simulink model "ofdm4"  (R2018b)
settings: Solver=VariableStepAuto  StartTime=0.0  StopTime=10.0  RelTol=1e-3
undefined symbols (not defined in the file or in its folder): doppler
libraries: commrandsrc3 x3, commutil2 x2, simulink x2, dspmathops x2, commdigbbndpm3 x2, commofdm x2, commrflib2 x2, commfilt2 x2, commdigbbndam3 x2, commsink2 x1, commchan3 x1
settings Model: Creator=Aviya  LastModifiedBy=Aviya

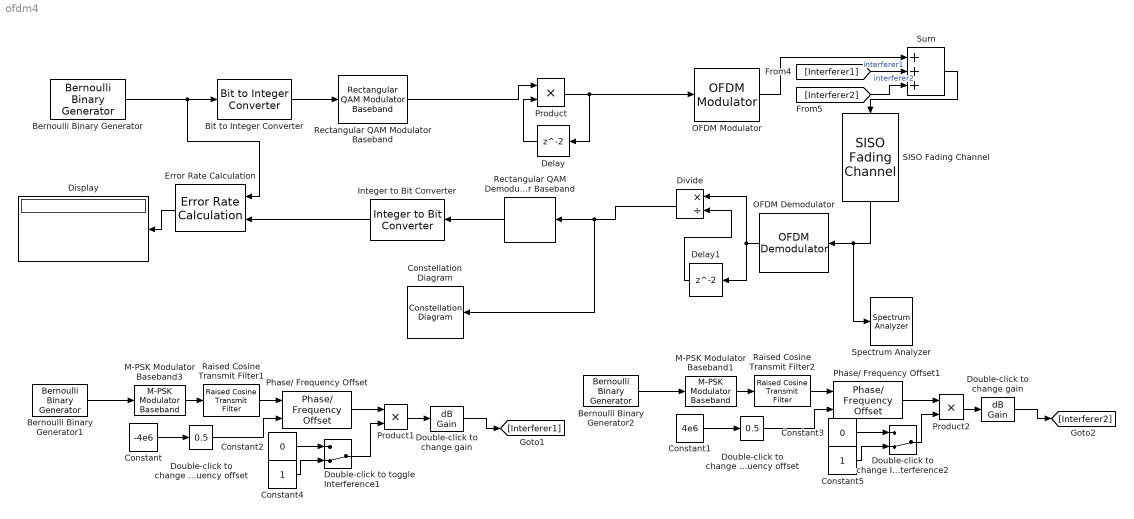
== system ofdm4 ==
  Bernoulli Binary Generator : commrandsrc3/Bernoulli Binary Generator  ProbabilityOfZero=0.5  SeedSource=Parameter  Seed=61  SampleTime=1  SamplesPerFrame=53  OutputDataType=double  SimulateUsing=Interpreted execution
      settings: SourceProductName=Communications Toolbox
  Bernoulli Binary Generator1 : commrandsrc3/Bernoulli Binary Generator  ProbabilityOfZero=0.5  SeedSource=Parameter  Seed=61  SampleTime=1  SamplesPerFrame=80  OutputDataType=boolean  SimulateUsing=Interpreted execution
  Bernoulli Binary Generator2 : commrandsrc3/Bernoulli Binary Generator  ProbabilityOfZero=0.5  SeedSource=Parameter  Seed=61  SampleTime=1  SamplesPerFrame=80  OutputDataType=boolean  SimulateUsing=Interpreted execution
  Bit to Integer Converter : commutil2/Bit to Integer Converter  nbits=1  bitOrder=MSB first  signedOutputValues=Unsigned  outDtype=single  outDtypeSigned=Inherit via internal rule
      settings: SourceProductName=Communications Toolbox
  Constant : Constant  Value=-4e6  VectorParams1D=off  SampleTime=(1e-6/3)*300
  Constant1 : Constant  Value=4e6  VectorParams1D=off  SampleTime=(1e-6/3)*300
  Constant2 : Constant  Value=0  VectorParams1D=off  SampleTime=(1e-6/3)*300
  Constant3 : Constant  Value=0  VectorParams1D=off  SampleTime=(1e-6/3)*300
  Constant4 : Constant  VectorParams1D=off  SampleTime=(1e-6/3)*300
  Constant5 : Constant  VectorParams1D=off  SampleTime=(1e-6/3)*300
  Constellation Diagram : ConstellationDiagram
  Delay : Delay
  Delay1 : Delay
  Display : Display
  Divide : Product  Inputs=*/
  Double-click to change Interference2 : ManualSwitch  CurrentSetting=0
  Double-click to change frequency offset : simulink/Math Operations/Slider Gain  gain=0.5  low=-0.85  high=0.85
  Double-click to change gain : dspmathops/dB Gain  dB=-20  intype=Amplitude
      settings: SourceProductName=DSP System Toolbox  SourceProductBaseCode=DS
  "Double-click to change gain " : dspmathops/dB Gain  dB=-10  intype=Amplitude
      settings: SourceProductName=DSP System Toolbox  SourceProductBaseCode=DS
  Double-click to toggle Interference1 : ManualSwitch  CurrentSetting=0
  Double-click to change frequency offset : simulink/Math Operations/Slider Gain  gain=0.5  low=-0.85  high=0.85
  Error Rate Calculation : commsink2/Error Rate Calculation  N=0  st_delay=0  cp_mode=Entire frame  subframe=[]  PMode=Port  WsName=ErrorVec  RsMode2=off  stop=off  numErr=100  maxBits=1e6
      settings: SourceProductName=Communications Toolbox
  Integer to Bit Converter : commutil2/Integer to Bit Converter  nbits=1  signedInputValues=Unsigned  bitOrder=MSB first  outDtype=Inherit via internal rule
      settings: SourceProductName=Communications Toolbox
  M-PSK Modulator Baseband1 : commdigbbndpm3/M-PSK Modulator Baseband  M=2  InType=Bit  Enc=Gray  Mapping=0  Ph=0  outDtype=double  outWordLen=16  outUDDataType=sfix(16)  outFracLenMode=Best precision  outFracLen=15  outDataTypeStr=double  outLastDataTypeStr=double
      settings: SourceProductName=Communications System Toolbox
  M-PSK Modulator Baseband3 : commdigbbndpm3/M-PSK Modulator Baseband  M=2  InType=Integer  Enc=Gray  Mapping=0  Ph=0  outDtype=double  outWordLen=16  outUDDataType=sfix(16)  outFracLenMode=Best precision  outFracLen=15  outDataTypeStr=double  outLastDataTypeStr=double
      settings: SourceProductName=Communications System Toolbox
  OFDM Demodulator : commofdm/OFDM Demodulator  FFTLength=64  NumGuardBandCarriers=[6; 5]  RemoveDCCarrier=off  PilotOutputPort=off  PilotCarrierIndices=[12; 26; 40; 54]  CyclicPrefixLength=16  NumSymbols=1  NumReceiveAntennas=1  SimulateUsing=Interpreted execution
      settings: SourceProductName=Communications Toolbox  SourceProductBaseCode=CM
  OFDM Modulator : commofdm/OFDM Modulator  FFTLength=64  NumGuardBandCarriers=[6;5]  InsertDCNull=off  PilotInputPort=off  PilotCarrierIndices=[12; 26; 40; 54]  CyclicPrefixLength=16  Windowing=off  WindowLength=1  NumSymbols=1  NumTransmitAntennas=1  SimulateUsing=Interpreted execution
      settings: SourceProductName=Communications Toolbox  SourceProductBaseCode=CM
  Phase/ Frequency Offset : commrflib2/Phase// Frequency Offset  phaseOffset=0  freqPort=on  freqOffset=0
      settings: SourceProductName=Communications System Toolbox
  Phase/ Frequency Offset1 : commrflib2/Phase// Frequency Offset  phaseOffset=0  freqPort=on  freqOffset=0
      settings: SourceProductName=Communications System Toolbox
  Product : Product
  Product1 : Product  SaturateOnIntegerOverflow=on  OutDataTypeStr=Inherit: Same as first input
  Product2 : Product  SaturateOnIntegerOverflow=on  OutDataTypeStr=Inherit: Same as first input
  Raised Cosine Transmit Filter1 : commfilt2/Raised Cosine Transmit Filter  filtType=Square root  R=0.22  filtSpan=12  N=2  filterGain=1  RateOptions=Allow multirate processing  framing=Mute  checkCoeff=off  variableName=rcTxFilt1  checkGain=Normalized  sampMode=Mute  saveAsFlag=0  currentFiltSpan=12  D=(12)/2  launchFVT=off  roundingMode=Floor  overflowMode=off  coeffDataTypeStr=Inherit: Same word length as input  coeffMin=[]  coeffMax=[]  coeffLastDataTypeStr=Inherit: Same word length as input  outputDataTypeStr=Inherit: Same as accumulator  outputMin=[]  outputMax=[]  outputLastDataTypeStr=Inherit: Same as accumulator
  Raised Cosine Transmit Filter2 : commfilt2/Raised Cosine Transmit Filter  filtType=Square root  R=0.22  filtSpan=12  N=2  filterGain=1  RateOptions=Allow multirate processing  framing=Mute  checkCoeff=off  variableName=rcTxFilt2  checkGain=Normalized  sampMode=Mute  saveAsFlag=0  currentFiltSpan=12  D=6  launchFVT=off  roundingMode=Floor  overflowMode=off  coeffDataTypeStr=Inherit: Same word length as input  coeffMin=[]  coeffMax=[]  coeffLastDataTypeStr=Inherit: Same word length as input  outputDataTypeStr=Inherit: Same as accumulator  outputMin=[]  outputMax=[]  outputLastDataTypeStr=Inherit: Same as accumulator
  Rectangular QAM Demodulator Baseband : commdigbbndam3/Rectangular QAM Demodulator Baseband  M=2  OutType=Integer  DecType=Hard decision  VarSource=Dialog  Variance=1  Dec=Gray  Mapping=[0:15]  PowType=Min. distance between symbols  MinDist=2  AvgPow=1  PeakPow=1  Ph=0  outDtype1=Inherit via internal rule  outDtype2=Inherit via internal rule  derotateFactorWordLen=16  derotateFactorDataTypeStr=Inherit: Same word length as input  derotateFactorLastDataTypeStr=Inherit: Same word length as input  denormFactorWordLen=16  denormFactorDataTypeStr=Inherit: Same word length as input  denormFactorLastDataTypeStr=Inherit: Same word length as input  prodOutWordLen=32  prodOutOverflowMode=Wrap  prodOutRoundingMode=Floor  prodOutOvFlMode=off  prodOutOvFlModeLastStrValue=off  sumWordLen=32
      settings: SourceProductName=Communications Toolbox
  Rectangular QAM Modulator Baseband : commdigbbndam3/Rectangular QAM Modulator Baseband  M=16  InType=Integer  Enc=Gray  Mapping=[0:15]  PowType=Average Power  MinDist=2  AvgPow=1  PeakPow=1  Ph=0  outDtype=double  outWordLen=32  outUDDataType=sfix(16)  outFracLenMode=Best precision  outFracLen=15  outDataTypeStr=double  outLastDataTypeStr=double
      settings: SourceProductName=Communications Toolbox
  SISO Fading Channel : commchan3/SISO Fading Channel  InheritSampleRate=on  SampleRate=1  PathDelays=0  AveragePathGains=0  NormalizePathGains=on  FadingDistribution=Rayleigh  KFactor=3  DirectPathDopplerShift=0  DirectPathInitialPhase=0  MaximumDopplerShift=0.001  DopplerSpectrum=doppler('Jakes')  ChannelInterpolationMethod=Polyphase  RandomStream=mt19937ar with seed  RandomNumGenerator=mt19937ar  Seed=73  PathGainsOutputPort=off  ChannelFilterDelayOutputPort=off  SimulateUsing=Interpreted execution  Visualization=Off  PathsForDopplerDisplay=1  SamplesToDisplay=25%
      settings: SourceProductName=Communications Toolbox
  Spectrum Analyzer : SpectrumAnalyzer
  Sum : Sum  Inputs=+++  SaturateOnIntegerOverflow=on
  wires:
  Bit to Integer Converter/1 -> Rectangular QAM Modulator Baseband/1
  Rectangular QAM Modulator Baseband/1 -> Product/1
  Delay/1 -> Product/2
  Product/1 -> OFDM Modulator/1, Delay/1
  Rectangular QAM Demodulator Baseband/1 -> Integer to Bit Converter/1
  OFDM Demodulator/1 -> Delay1/1, Divide/1
  Delay1/1 -> Divide/2
  Integer to Bit Converter/1 -> Error Rate Calculation/2
  Error Rate Calculation/1 -> Display/1
  Bernoulli Binary Generator/1 -> Bit to Integer Converter/1, Error Rate Calculation/1
  SISO Fading Channel/1 -> Spectrum Analyzer/1, OFDM Demodulator/1
  M-PSK Modulator Baseband1/1 -> Raised Cosine Transmit Filter2/1
  Bernoulli Binary Generator1/1 -> M-PSK Modulator Baseband3/1
  M-PSK Modulator Baseband3/1 -> Raised Cosine Transmit Filter1/1
  Constant2/1 -> Double-click to toggle Interference1/1
  Product2/1 -> "Double-click to change gain "/1
  Double-click to change frequency offset/1 -> Phase/ Frequency Offset/2
  Double-click to change Interference2/1 -> Product2/2
  Constant/1 -> Double-click to change frequency offset/1
  "Double-click to change gain "/1 -> [Interferer2]
  Constant3/1 -> Double-click to change Interference2/1
  Double-click to toggle Interference1/1 -> Product1/2
  Constant1/1 -> Double-click to change frequency offset/1
  [Interferer1] -> Sum/2  "interferer1"
  Constant5/1 -> Double-click to change Interference2/2
  Raised Cosine Transmit Filter1/1 -> Phase/ Frequency Offset/1
  Bernoulli Binary Generator2/1 -> M-PSK Modulator Baseband1/1
  Double-click to change frequency offset/1 -> Phase/ Frequency Offset1/2
  Phase/ Frequency Offset1/1 -> Product2/1
  Constant4/1 -> Double-click to toggle Interference1/2
  Raised Cosine Transmit Filter2/1 -> Phase/ Frequency Offset1/1
  Phase/ Frequency Offset/1 -> Product1/1
  Double-click to change gain/1 -> [Interferer1]
  Product1/1 -> Double-click to change gain/1
  Divide/1 -> Constellation Diagram/1, Rectangular QAM Demodulator Baseband/1
  OFDM Modulator/1 -> Sum/1
  Sum/1 -> SISO Fading Channel/1
  [Interferer2] -> Sum/3  "interferer2"
